simulink model "observer_LQR"  (R2024b)
settings: Solver=VariableStepAuto  StartTime=0.0  StopTime=10.0  RelTol=1e-3
values from neighbouring files (symbols this model uses):
  A = output{1}    [task3.m]
  B = output{2}    [task3.m]
  C = output{3}    [task3.m]
  K = R\B'*P    [task3.m]
  L = K_tilde'    [task3.m]
  x_0 = output{5}    [task3.m]
settings Model: Creator=wyton  LastModifiedBy=KevinNuo
settings SolverCC: AlgebraicLoopSolver=TrustRegion
settings OptimizationCC: ReuseModelBlockBuffer=off
settings DebuggingCC: UnconnectedInputMsg=warning  UnconnectedOutputMsg=warning  UnconnectedLineMsg=warning
settings ModelReferenceCC: EnableRefExpFcnMdlSchedulingChecks=on
settings RTWCC: GPUComputeCapability=3.5  DLArmComputeVersion=19.05

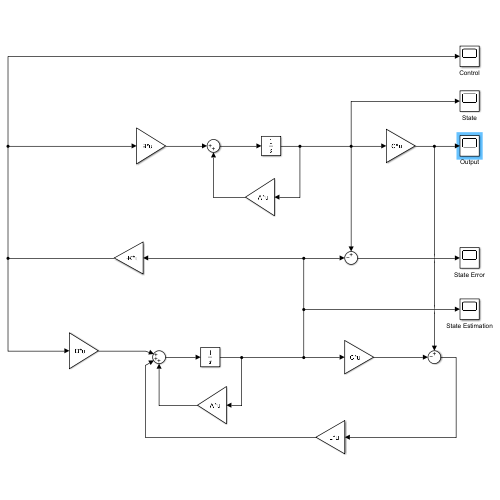
[thumbnail: Simulink's stored preview of the top-level diagram]
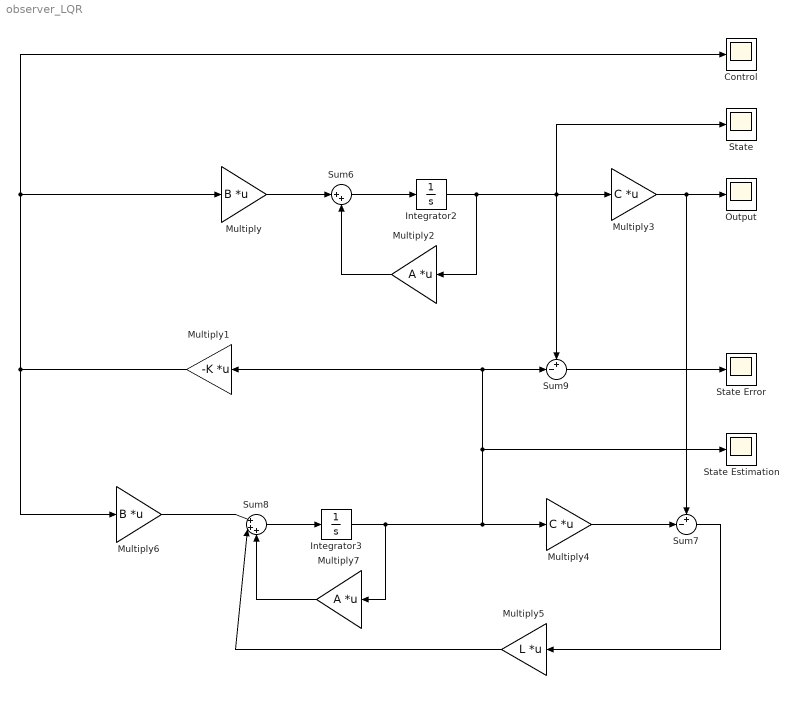
== system observer_LQR ==
  Control : Scope
  Integrator2 : Integrator  InitialCondition=x_0
  Integrator3 : Integrator
  Multiply : Gain  Gain=B  Multiplication=Matrix(K*u)
  Multiply1 : Gain  Gain=-K  Multiplication=Matrix(K*u)
  Multiply2 : Gain  Gain=A  Multiplication=Matrix(K*u)
  Multiply3 : Gain  Gain=C  Multiplication=Matrix(K*u)
  Multiply4 : Gain  Gain=C  Multiplication=Matrix(K*u)
  Multiply5 : Gain  Gain=L  Multiplication=Matrix(K*u)
  Multiply6 : Gain  Gain=B  Multiplication=Matrix(K*u)
  Multiply7 : Gain  Gain=A  Multiplication=Matrix(K*u)
  Output : Scope
  State : Scope
  State Error : Scope
  State Estimation : Scope
  Sum6 : Sum  Inputs=|++
  Sum7 : Sum  Inputs=+-|
  Sum8 : Sum  Inputs=|+++
  Sum9 : Sum  Inputs=+-|
  wires:
  Sum6/1 -> Integrator2/1
  Multiply/1 -> Sum6/1
  Multiply2/1 -> Sum6/2
  Multiply3/1 -> Sum7/1, Output/1
  Integrator2/1 -> State/1, Sum9/1, Multiply3/1, Multiply2/1
  Multiply4/1 -> Sum7/2
  Sum7/1 -> Multiply5/1
  Integrator3/1 -> Multiply1/1, Sum9/2, State Estimation/1, Multiply4/1, Multiply7/1
  Multiply6/1 -> Sum8/1
  Sum8/1 -> Integrator3/1
  Multiply7/1 -> Sum8/3
  Multiply5/1 -> Sum8/2
  Sum9/1 -> State Error/1
  Multiply1/1 -> Control/1, Multiply/1, Multiply6/1
